simulink subsystem "Trigger_Regulator"  (R2023a)
settings: Solver=VariableStepAuto  StartTime=0.0  StopTime=10.0  RelTol=1e-3
settings Model: Creator=user  LastModifiedBy=user

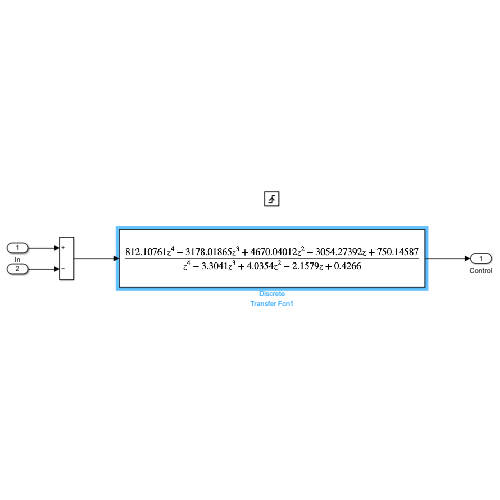
[thumbnail: Simulink's stored preview of the top-level diagram]
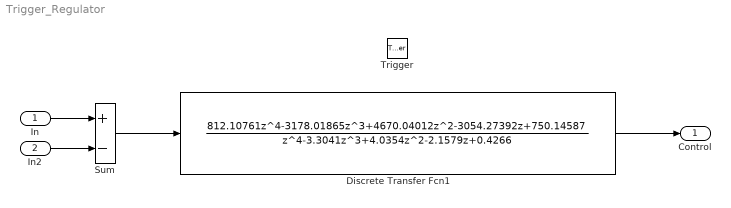
== system Trigger_Regulator ==
  In : Inport
  In2 : Inport  Port=2
  Trigger : TriggerPort  VariantControl=(inherit)  PortDimensions=1
  Discrete Transfer Fcn1 : DiscreteTransferFcn  Numerator=[812.10761, -3178.01865, 4670.04012, -3054.27392, 750.14587 ]  Denominator=[1, -3.3041, 4.0354, -2.1579, 0.4266]
  Sum : Sum  Inputs=+-
  Control : Outport
  wires:
  Sum/1 -> Discrete Transfer Fcn1/1
  In2/1 -> Sum/2
  In/1 -> Sum/1
  Discrete Transfer Fcn1/1 -> Control/1
